simulink model "TST_StateflowBitOperations"  (Simulink 7.8)
settings: Solver=FixedStepDiscrete  StartTime=0.0  StopTime=10.0  FixedStep=0.02  RelTol=1e-3
settings Model: Creator=kharthforeign  LastModifiedBy=kharthforeign  BufferReuse=off
settings DataIOCC: SaveOutput=off  SignalLogging=off  SaveTime=off
settings OptimizationCC: BlockReduction=off  ConditionallyExecuteInputs=off  OptimizeBlockIOStorage=off  BufferReuse=off  ExpressionFolding=off  LocalBlockOutputs=off  InitFltsAndDblsToZero=on
settings DebuggingCC: FcnCallInpInsideContextMsg=Use local settings  StrictBusMsg=Warning

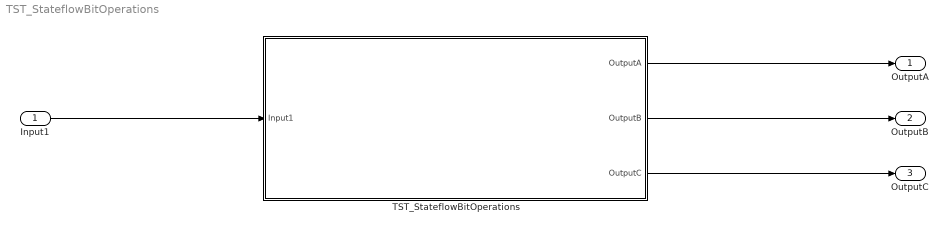
== system TST_StateflowBitOperations ==
  Input1 : Inport  OutDataTypeStr=uint32  BusOutputAsStruct=on
  TST_StateflowBitOperations : Subsystem  TreatAsAtomicUnit=on
  OutputA : Outport  OutDataTypeStr=double  PortDimensions=1
  OutputB : Outport  Port=2  OutDataTypeStr=double  PortDimensions=1
  OutputC : Outport  Port=3  OutDataTypeStr=double  PortDimensions=1
  wires:
  Input1/1 -> TST_StateflowBitOperations/1(Input1)
  TST_StateflowBitOperations/1(OutputA) -> OutputA/1
  TST_StateflowBitOperations/2(OutputB) -> OutputB/1
  TST_StateflowBitOperations/3(OutputC) -> OutputC/1

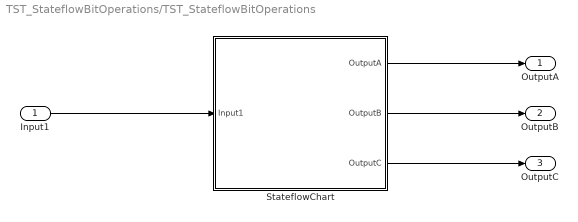
== system TST_StateflowBitOperations/TST_StateflowBitOperations ==
  Input1 : Inport  OutDataTypeStr=uint32  BusOutputAsStruct=on
  StateflowChart : Stateflow chart  TreatAsAtomicUnit=on
  OutputA : Outport  OutDataTypeStr=double  PortDimensions=1
  OutputB : Outport  Port=2  OutDataTypeStr=double  PortDimensions=1
  OutputC : Outport  Port=3  OutDataTypeStr=double  PortDimensions=1
  wires:
  StateflowChart/1(OutputA) -> OutputA/1
  StateflowChart/2(OutputB) -> OutputB/1
  StateflowChart/3(OutputC) -> OutputC/1
  Input1/1 -> StateflowChart/1(Input1)

== stateflow chart TST_StateflowBitOperations/StateflowChart ==
  state DummyState
    entry:
    % reset CrcValue
    CrcValue = uint16(0);
    % feed first byte
    CrcValue = UpdateCrc16(CrcValue, uint8(123));
    % feed second byte
    CrcValue = UpdateCrc16(CrcValue, uint8(234));
    % feed third byte, etc...
    CrcValue = UpdateCrc16(CrcValue, uint8(234));
    % split the resultinh uint16 CrcValue into uint8 high and low byte
    CrcBytes[uint32(0)] = (uint16(65280) & CrcValue) >> uint32(8);
    CrcBytes[uint32(1)] = uint16(255) & CrcValue;
  state CrcResult = UpdateCrc16(CrcStartValue, CurrentByte) [function]
    (default) -> (junction 5)
    (junction 5) -> (junction 6) : {...
        |    TableIndex = ((CrcStartValue >> uint32(8)) ^ CurrentByte);...
        |    CrcResult = uint16(((CrcStartValue << uint32(8)) ^ GBL_ChecksumUtil_DataTable16[TableIndex]));...
        | }
  (default) -> DummyState
  data: CrcStartValue function_input uint16; CurrentByte function_input uint8; CrcResult function_output uint16; TableIndex temporary uint16; Input1 input uint32; OutputA output double =1; OutputB output double =2; OutputC output double =3; CrcValue local uint16 =0; GBL_ChecksumUtil_DataTable16 constant uint16 size=256 =TST_CrcTable_Data; CrcBytes local uint8 size=2
